simulink model "simulation_64_apsk"  (R2025b)
settings: Solver=VariableStepAuto  StartTime=0.0  StopTime=1e-5  RelTol=1e-3
undefined symbols (not defined in the file): PSK
libraries: commfilt2 x2, commdigbbndapm x1, commrandsrc3 x1
settings Model: Creator=Panos  LastModifiedBy=Panos

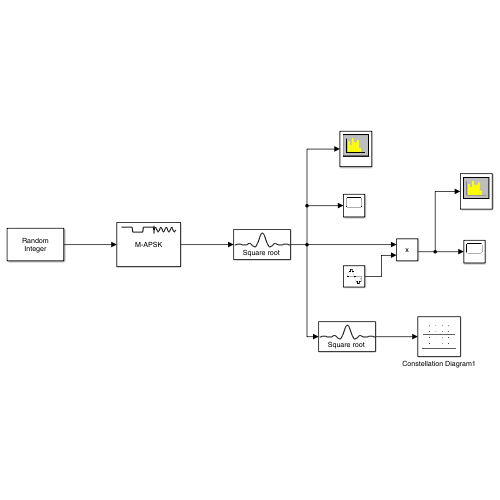
[thumbnail: Simulink's stored preview of the top-level diagram]
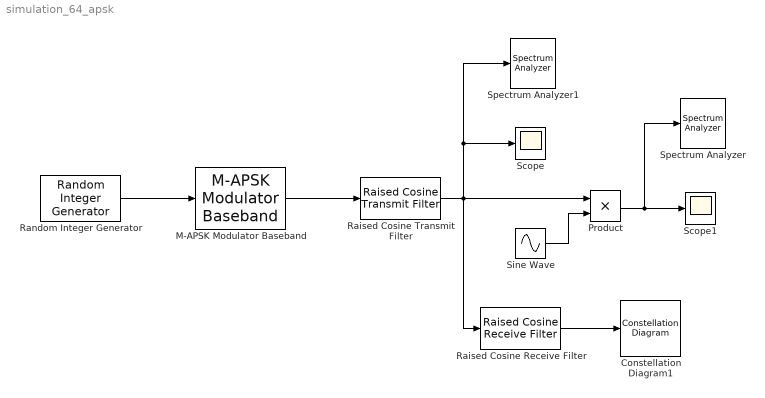
== system simulation_64_apsk ==
  Constellation Diagram1 : ConstellationDiagram  WindowPosition=[1.000000,49.000000,2048.000000,1081.000000,]  ScopeFrameLocation=window  SamplesPerSymbol=8  SymbolsToDisplaySource=Property  SymbolsToDisplay=1000  ReferenceConstellation=8-PSK  ShowLegend=on  ShowReferenceConstellation=off
  M-APSK Modulator Baseband : commdigbbndapm/M-APSK Modulator Baseband  ConstPointsCirclewise=[4, 12, 20, 28]  Radii=[1, 2.4, 4.3, 7]  PhaseOffset=mod([pi/4, pi/12, 3*pi/20, 13*pi/28], 2*pi./[4, 12, 20, 28])  SymbolMapping=Auto  CustomSymbolMapping=[ 0, 4, 12, 8, 1, 3, 2, 6, 7, 5, 13, 15, 14, 10, 11, 9 ]  InputType=Integer  OutputDataType=double  SimulateUsing=Code generation
  Product : Product
  Raised Cosine Receive Filter : commfilt2/Raised Cosine Receive Filter  filtType=Square root  R=0.2  filtSpan=16  N=8  downFactor=8  downOffset=0  filterGain=1  InputProcessing=Columns as channels (frame based)  RateOptions=Allow multirate processing  framing=Mute  checkCoeff=off  variableName=rcRxFilt  currentFiltSpan=10  D=5  inputOffset=0  sampMode=Mute  saveAsFlag=0  rateMode=Downsampling  checkGain=Normalized  launchFVT=on  roundingMode=Floor  overflowMode=off  coeffDataTypeStr=Inherit: Same word length as input  coeffMin=[]  coeffMax=[]  coeffLastDataTypeStr=Inherit: Same word length as input  accumDataTypeStr=Inherit: Same as product output  accumLastDataTypeStr=Inherit: Same as product output  outputDataTypeStr=Inherit: Same as accumulator  outputMin=[]  outputMax=[]  outputLastDataTypeStr=Inherit: Same as accumulator
  Raised Cosine Transmit Filter : commfilt2/Raised Cosine Transmit Filter  filtType=Square root  R=0.2  filtSpan=16  N=8  filterGain=1  InputProcessing=Columns as channels (frame based)  RateOptions=Allow multirate processing  framing=Mute  checkCoeff=off  variableName=rcTxFilt  checkGain=Normalized  sampMode=Mute  saveAsFlag=0  currentFiltSpan=10  D=(10)/2  launchFVT=on  roundingMode=Floor  overflowMode=off  coeffDataTypeStr=Inherit: Same word length as input  coeffMin=[]  coeffMax=[]  coeffLastDataTypeStr=Inherit: Same word length as input  outputDataTypeStr=Inherit: Same as accumulator  outputMin=[]  outputMax=[]  outputLastDataTypeStr=Inherit: Same as accumulator
  Random Integer Generator : commrandsrc3/Random Integer Generator  SetSize=64  SeedSource=Auto  Seed=0  SampleTime=8e-9  SamplesPerFrame=1  OutputDataType=double  SimulateUsing=Interpreted execution
  Scope : Scope
      settings: ActiveDisplayYMinimum=-7.6567263307793176  ActiveDisplayYMaximum=7.8302436061956291
  Scope1 : Scope
      settings: ActiveDisplayYMinimum=-7.1137650990564758  ActiveDisplayYMaximum=9.1462694130779862
  Sine Wave : Sin  Frequency=2*pi*24.125e9  SampleTime=1e-11
  Spectrum Analyzer : SpectrumAnalyzer  WindowPosition=[1.000000,49.000000,2048.000000,1081.000000,]  ScopeFrameLocation=window  PlotAsTwoSidedSpectrum=off  WindowInvariantSamplesPerUpdate=on  NumTapsPerBand=38  FilterSharpness=0.8  FrequencySpan=Span and center frequency  Span=10e9  CenterFrequency=24.125e9  StartFrequency=0  ReferenceLoad=50  YLimits=[-101.7282 17.5749]
  Spectrum Analyzer1 : SpectrumAnalyzer  WindowPosition=[1.000000,49.000000,2048.000000,1081.000000,]  ScopeFrameLocation=window  PlotAsTwoSidedSpectrum=off  WindowInvariantSamplesPerUpdate=on  NumTapsPerBand=38  FilterSharpness=0.8  FrequencySpan=Span and center frequency  Span=10e9  CenterFrequency=24.125e9  StartFrequency=0  ReferenceLoad=50  YLimits=[-101.7282 17.5749]
  wires:
  Random Integer Generator/1 -> M-APSK Modulator Baseband/1
  Sine Wave/1 -> Product/2
  Product/1 -> Spectrum Analyzer/1, Scope1/1
  M-APSK Modulator Baseband/1 -> Raised Cosine Transmit Filter/1
  Raised Cosine Transmit Filter/1 -> Spectrum Analyzer1/1, Scope/1, Product/1, Raised Cosine Receive Filter/1
  Raised Cosine Receive Filter/1 -> Constellation Diagram1/1
